simulink model "Aries"  (R2026a)
settings: Solver=VariableStepAuto
undefined symbols (not defined in the file): physconst
libraries: phasedenvlib x4, phasedtxrxlib x3, dspstat3 x1, phasedbflib x1
settings Model: Creator=Anunnya  LastModifiedBy=Anunnya

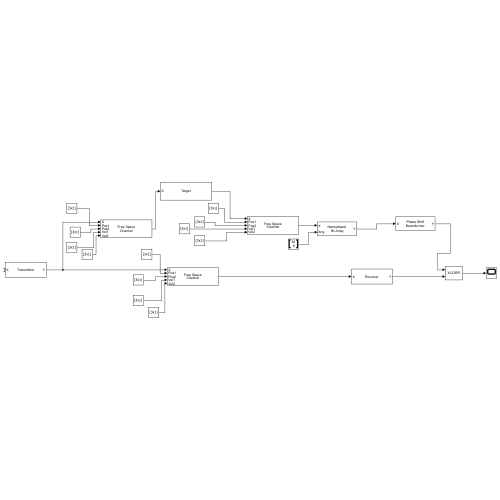
[thumbnail: Simulink's stored preview of the top-level diagram]
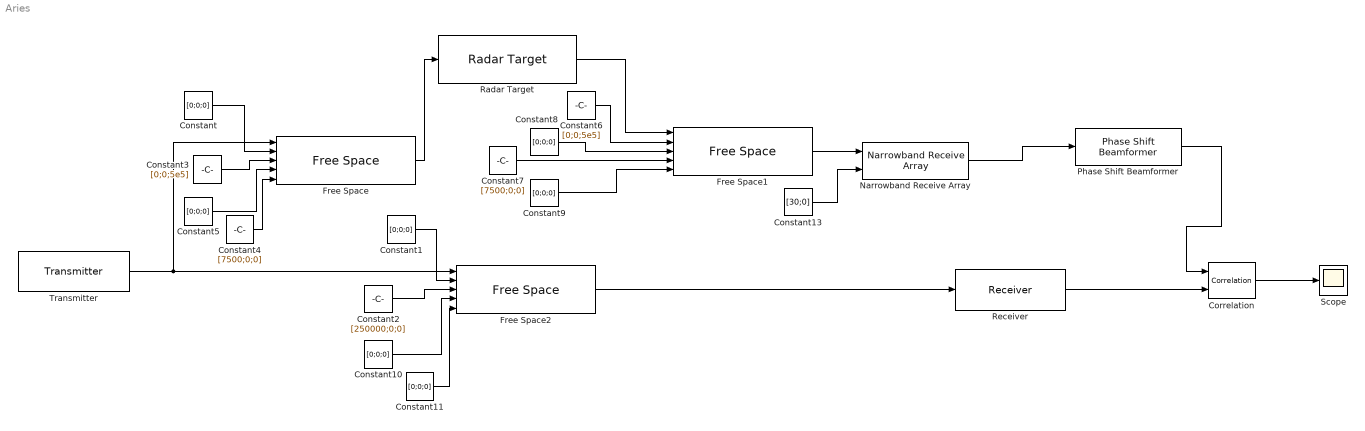
== system Aries ==
  Constant : Constant  Value=[0;0;0]
  Constant{1,8..11} (5 alike) : Constant  Value=[0;0;0]  VectorParams1D=off
  Constant13 : Constant  Value=[30;0]  VectorParams1D=off
  Constant2 : Constant  Value=[250000;0;0]  VectorParams1D=off
  Constant3 : Constant  Value=[0;0;5e5]
  Constant4 : Constant  Value=[7500;0;0]
  Constant5 : Constant  Value=[0;0;0]
  Constant6 : Constant  Value=[0;0;5e5]  VectorParams1D=off
  Constant7 : Constant  Value=[7500;0;0]  VectorParams1D=off
  Correlation : dspstat3/Correlation  domain=Time  roundingMode=Floor  overflowMode=off  outputDataTypeStr=Inherit: Same as accumulator  outputMin=[]  outputMax=[]  outputLastDataTypeStr=Inherit: Same as accumulator
  Free Space : phasedenvlib/Free Space  PropagationSpeed=physconst( 'LightSpeed' )  OperatingFrequency=206.5e6  TwoWayPropagation=off  SampleRateFromInputCheckbox=on  SampleRate=1e6  MaximumDistanceSource=Property  MaximumDistance=2e6  MaximumNumInputSamplesSource=Auto  MaximumNumInputSamples=1000  FractionalDelayMethod=Linear  SimulateUsing=Interpreted execution
  Free Space1 : phasedenvlib/Free Space  PropagationSpeed=physconst( 'LightSpeed' )  OperatingFrequency=206.5e6  TwoWayPropagation=off  SampleRateFromInputCheckbox=on  SampleRate=1e6  MaximumDistanceSource=Property  MaximumDistance=2e6  MaximumNumInputSamplesSource=Auto  MaximumNumInputSamples=1000  FractionalDelayMethod=Linear  SimulateUsing=Interpreted execution
  Free Space2 : phasedenvlib/Free Space  PropagationSpeed=physconst( 'LightSpeed' )  OperatingFrequency=206.5e6  TwoWayPropagation=off  SampleRateFromInputCheckbox=on  SampleRate=1e6  MaximumDistanceSource=Property  MaximumDistance=2e6  MaximumNumInputSamplesSource=Auto  MaximumNumInputSamples=1000  FractionalDelayMethod=Linear  SimulateUsing=Interpreted execution
  Narrowband Receive Array : phasedtxrxlib/Narrowband Receive Array  PropagationSpeed=physconst( 'LightSpeed' )  OperatingFrequency=206.5e6  Wavefront=Plane  SensorGainMeasure=dB  Polarization=None  WeightsInputPort=off  SimulateUsing=Interpreted execution  Sensor=|
      | phased.ConformalArray(ElementPosition=[ 0        0.726    0.363   -0.363   -0.726   -0.363    0.363;
      |   0        0        0.629    0.629    0       -0.629   -0.629;
      |   0        0        0        0        0        0        0],Element=phased.IsotropicAntennaElement())
  Phase Shift Beamformer : phasedbflib/Phase Shift Beamformer  PropagationSpeed=physconst( 'LightSpeed' )  OperatingFrequency=206.5e6  DirectionSource=Property  Direction=[ 30; 0 ]  NumPhaseShifterBits=0  WeightsNormalization=Distortionless  WeightsOutputPort=off  SimulateUsing=Interpreted execution  SensorArray=|
      | phased.ConformalArray(ElementPosition=[ 0        0.726    0.363   -0.363   -0.726   -0.363    0.363;
      |   0        0        0.629    0.629    0       -0.629   -0.629;
      |   0        0        0        0        0        0        0],Element=phased.IsotropicAntennaElement())
  Radar Target : phasedenvlib/Radar Target  EnablePolarization=off  Mode=Monostatic  MeanRCSSource=Property  ScatteringMatrixSource=Property  MeanRCS=1  ScatteringMatrix=eye( 2 )  Model=Nonfluctuating  PropagationSpeed=physconst( 'LightSpeed' )  OperatingFrequency=206.5e6  SeedSource=Auto  Seed=0  SimulateUsing=Interpreted execution
  Receiver : phasedtxrxlib/Receiver  Configuration=Budget  EnableInputPort=off  SampleRate=1e6  SampleRateFromInputCheckbox=on  SimulateUsing=Interpreted execution  GainMethod=Linear  Gain=10  OIP3=Inf  Table=[ -25, 5, -1; -10, 20, -2; 0, 27, 12; 5, 28, 12 ]  NoiseMethod=Noise figure  NoiseFigure=3  NoiseFactor=2  NoiseTemperature=290  ReferenceTemperature=290  PhaseOffset=0  AddInputNoise=on  InputNoiseTemperature=290  SeedSource=Auto  Seed=0
  Scope : Scope
  Transmitter : phasedtxrxlib/Transmitter  Configuration=EIRP  InUseOutputPort=off  CoherentOnTransmit=on  PhaseNoiseOutputPort=off  SampleRate=1e6  SampleRateFromInputCheckbox=on  SimulateUsing=Interpreted execution  PeakPower=235000  GainMethod=Linear  Gain=34  LossFactor=0  OIP3=Inf  Table=[ -25, 5, -1; -10, 20, -2; 0, 27, 12; 5, 28, 12 ]  NoiseMethod=None  NoiseFigure=0  NoiseFactor=1  NoiseTemperature=0  ReferenceTemperature=290  PhaseOffset=0  SeedSource=Auto  Seed=0
  wires:
  Free Space/1 -> Radar Target/1
  Radar Target/1 -> Free Space1/1
  Transmitter/1 -> Free Space2/1, Free Space/1
  Receiver/1 -> Correlation/2
  Free Space1/1 -> Narrowband Receive Array/1
  Phase Shift Beamformer/1 -> Correlation/1
  Constant/1 -> Free Space/2
  Free Space2/1 -> Receiver/1
  Constant1/1 -> Free Space2/2
  Constant2/1 -> Free Space2/3
  Constant3/1 -> Free Space/3
  Constant4/1 -> Free Space/5
  Constant5/1 -> Free Space/4
  Constant6/1 -> Free Space1/2
  Constant7/1 -> Free Space1/4
  Constant8/1 -> Free Space1/3
  Constant9/1 -> Free Space1/5
  Correlation/1 -> Scope/1
  Constant10/1 -> Free Space2/4
  Constant11/1 -> Free Space2/5
  Narrowband Receive Array/1 -> Phase Shift Beamformer/1
  Constant13/1 -> Narrowband Receive Array/2
